simulink model "untitled"  (R2023a)
settings: Solver=VariableStepAuto  StartTime=0.0  StopTime=10.0  RelTol=1e-3
settings Model: Creator=s3928  LastModifiedBy=s3928

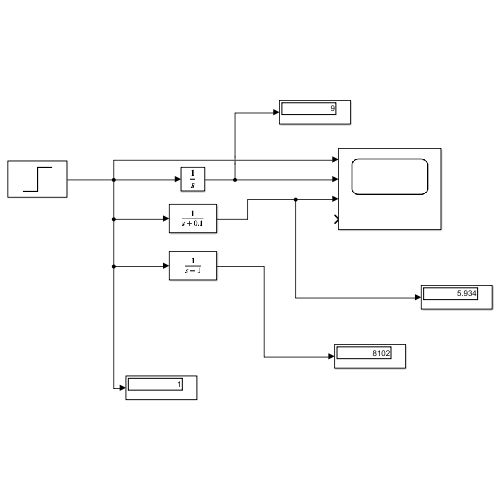
[thumbnail: Simulink's stored preview of the top-level diagram]
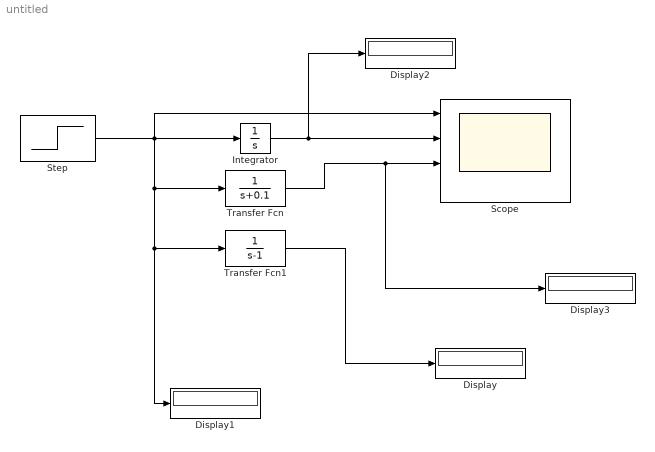
== system untitled ==
  Display{,1..3} (4 alike) : Display
  Integrator : Integrator
  Scope : Scope  NumInputPorts=4
  Step : Step  SampleTime=0
  Transfer Fcn : TransferFcn  Denominator=[1 0.1]
  Transfer Fcn1 : TransferFcn  Denominator=[1 -1]
  wires:
  Step/1 -> Integrator/1, Scope/1, Transfer Fcn1/1, Display1/1, Transfer Fcn/1
  Integrator/1 -> Display2/1, Scope/2
  Transfer Fcn1/1 -> Display/1
  Transfer Fcn/1 -> Display3/1, Scope/3
